simulink library "qs_model"  (R2016a)
settings: Solver=ode45  StartTime=0.0  StopTime=10.0  RelTol=1e-3
values from neighbouring files (symbols this model uses):
  step_time = 0.005    [initialize_variables_kuramoto.m]
libraries: simulink x2
settings Model: Creator=Kundan Panta  LastModifiedBy=Kundan Panta
settings DataIOCC: LimitDataPoints=on
settings DebuggingCC: AllowSymbolicDim=off

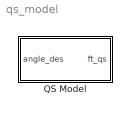
== system qs_model ==
  QS Model : Subsystem

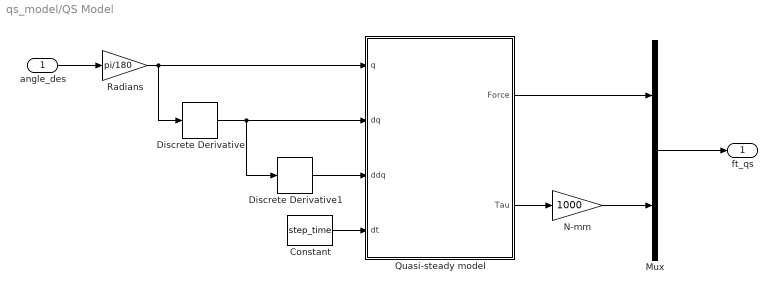
== system qs_model/QS Model ==
  angle_des : Inport  PortDimensions=3
  Constant : Constant  Value=step_time
  Discrete Derivative : simulink/Discrete/Discrete Derivative  gainval=1.0  ICPrevScaledInput=0.0  OutMin=[]  OutMax=[]  OutDataType=fixdt(1, 16)  OutScaling=2^-10  DoSatur=off
  Discrete Derivative1 : simulink/Discrete/Discrete Derivative  gainval=1.0  ICPrevScaledInput=0.0  OutMin=[]  OutMax=[]  OutDataType=fixdt(1, 16)  OutScaling=2^-10  DoSatur=off
  Mux : Mux  Inputs=2
  N-mm : Gain  Gain=1000
  Quasi-steady model : MATLAB Function  TreatAsAtomicUnit=on
  Radians : Gain  Gain=pi/180
  ft_qs : Outport
  wires:
  Quasi-steady model/1(Force) -> Mux/1
  Radians/1 -> Discrete Derivative/1, Quasi-steady model/1(q)
  Quasi-steady model/2(Tau) -> N-mm/1
  Mux/1 -> ft_qs/1
  Constant/1 -> Quasi-steady model/4(dt)
  Discrete Derivative/1 -> Quasi-steady model/2(dq), Discrete Derivative1/1
  angle_des/1 -> Radians/1
  Discrete Derivative1/1 -> Quasi-steady model/3(ddq)
  N-mm/1 -> Mux/2

== matlab function qs_model/QS Model/Quasi-steady model ==
  data: q input; Force output; dq input; ddq input; dt input; Tau output
%#codegen

%%%%%%%%%%%%%%%%%%%%%%%%%%%%%%%%%%%%%%%%%%%%%%%%%%%%%%%%%%%%%%%%%%%%%%%%%%%
%%%%%%%%%%%%%%   Aerodynamic forces and moments calculator   %%%%%%%%%%%%%%
%%%%%%%%%%%%%%%%%%%%%%%%%%%%%%%%%%%%%%%%%%%%%%%%%%%%%%%%%%%%%%%%%%%%%%%%%%%

% This program calcuates the aerodynamic forces and moments generated by a
% flapping wing

% The aerodynamic forces and torques at each wing blade element is
% evaluated by aerodynamics

function [Force,Tau] =Aerodynamic_Force_Torque(q,dq,ddq,dt)
    
% q=[stroke angle;deviation angle; rotation angle]
% dq= dq/dt;
% ddq= dq/dt;

%% Define variables 
    
%     omega_l            % Anular velocity of wing in global frame
%     omega_l_d          % Anular Acc of Right wing in body frame
%     Rcl                %(Rcl* vector_follower=vector_base //    follwer is Wing and Global is base)

    [Rcl,omega_l,omega_l_d] = AngKinZXY(q,dq,ddq);
    %% Hinge parameters

%     lhz  --> Stroke Hinge offset in stroke frame
%     lhx  --> Deviation Hinge offset in deviation frame
%     lhy  --> Rotation Hinge offset in Rotation frame

% Change these parameter according to your setup 
    lhz = [0;0;0];
    lhx = [0;0;0];
    lhy = [0;0.051;0];
    

    vel_h_l = rotz(q(1))*( cross([0;0;dq(1)],lhz) + rotx(q(2))*( cross([dq(2);0;0],lhx) + roty(q(3))*cross([0;dq(3);0],lhy) ));       % Velocity of Hinge in global frame
    
    %% Transform to wing frame
 
    omega_l=Rcl\omega_l;
    omega_l_d=Rcl\omega_l_d;
    vel_h_l  =  Rcl\vel_h_l;
    % transform from global to wing frame



    %%
    rho = 826;      % air density  1.2041(20C) 1.1839(25C)  1.1644(30C)  1.455(35C)
    NumBlade = 10;         % spatial resolution: number of blade elements


% Change these parameter according to your setup 
    Rw = 0.15;          % wing length
    AR = 3;             % Aspect Ratio
    chord = Rw/AR;        % chord length
        

    %% step through a wing span: spanwise location: 0<i<=1
    
    % Initialise variables
    F_t = zeros(3,1);
    Tau_t = zeros(3,1);

    
    for j = 1:NumBlade
        i = j/NumBlade;
        
        % obtain local aerodynamic force/torques in Hinge frame
        % omega_l and omega_r; omega_l_d and omega_r_d in body frame
        % omega_b and vel_h are in global frame
        % omega_b and vel_h have to be expressed differently for left and right wings
        
        % Force and Torque at each blade elements
        [Fi_t, Taui_t] = aerodynamics_left(omega_l,vel_h_l,omega_l_d,i,dt,Rw,chord, NumBlade,rho);

       %% Summation along wing span
       % integrate along wing span and transform to stroke plane frame
       F_t = F_t +  Fi_t;    
       Tau_t =  Tau_t +  Taui_t;


    end

%     % All the forces and torque obtain are in Left and Right Wing frame
%     % Tranform them to Hinge frame 
%  
%     Force=Rcl*F_t;
% 
%     Tau=Rcl*Tau_t ;

    % Keep forces and torques in Wing frame rather than Hinge frame
    Force=F_t;
    Tau=Tau_t;
    
end





%% %%%%%%%%%%%%%%%%%%%%%%%%%%%%%%%%%%%%%%%%%%%%%%%%%%%%%%%%%%%%%%%%%%%%%%%%
%  %%%%%%%%%%%%%%%%%%%%%%%%%%%%%%%%%%%%%%%%%%%%%%%%%%%%%%%%%%%%%%%%%%%%%%%%
%  %%%%%%%%%%%%%%%%%%%%%%%%%%%%%%%%%%%%%%%%%%%%%%%%%%%%%%%%%%%%%%%%%%%%%%%%

%-------------------------------------------------------------------
%----------   Aerodynamics Module For Wing  -------------------
%-------------------------------------------------------------------

% This function takes in wing kinematics (angle/velocity/accleration) and body velocity
% and calcuates the aerodynamic force/torque created by each wing blade (w.r.t local blade coordinate frame)
% then convert it to Hinge frame

% torques are with respect to the wing hinges.

% all the values are w.r.t to local blade coordinate frame (different from stroke
% plane frame), except original input of vel_h, omega_w, omege_w_d and omega_b are in stroke plane frame

% wing coordinate frame: (left wing) x points to ventral side (normal to the wing surface), y from wing base to tip, z from trailing to leading edge

% export tip velocity and span-averaged angle of attack

function [Fi, Taui] = aerodynamics_left(omega_w,vel_h, omega_w_d,i,dt,Rw,chord, NumBlade,rho)
 

%% blade-element analysis 
    % i=location of the blade element
    rle = -i*Rw;  % spanwise location of the blade element
    
    % local wing blade velocity 
    vle = cross(omega_w,[0 rle 0]') + vel_h;            % local leading edge velocity in wing frame
    vle(2)=0;                                                   % igonre radial velocity component                                    

    % angular velocity of the last time instant, here omega_b is assumed to be constant
    omega_wLI = omega_w-omega_w_d*dt;
    
    % velocity of the last time instant
    
    vleLI = cross(omega_wLI,[0 rle 0]') + vel_h;                        
    vleLI(2)=0;                                                 % igonre radial velocity component   
    
    % linear accleration along xw direction
    acc_xw = (vle(1)-vleLI(1))/dt;
    % angualr acceleration about yw direction
    omega_yw_dot = omega_w_d(2);

    
    %% Direction of blade velocity
    % get the direction of the local blade velocity
    if norm(vle) ~= 0
        dir_vle = vle/norm(vle)  ;                 % local leading edge velocity direction vector in left wing frame
        alpha = abs(atan(dir_vle(1)/dir_vle(3)));  
    else
        dir_vle = [0;0;0];
        alpha = 0;  
    end
    
    % local drag direction
    dir_drag = -dir_vle;  
    dir_drag(2)=0; 
    % local lift direction
    dir_lift = roty( -sign( vle(1)) *pi/2 ) * dir_vle;         
    % local angle of attack (consider X as imaginary axis and Z as real axis, only 1st and 2nd quadrants are considered)

    %%  wing sectional lift and drag due to translational force components
    % (2*CD(alpha_l)*rle/R) is sectional drag coefficient
    q   = 0.5*rho*(norm(vle))^2;
    FDi = q*(CD_hu(alpha)) * chord * (Rw/NumBlade)*dir_drag;  
    FLi = q*(CL_hu(alpha)) * chord * (Rw/NumBlade)*dir_lift;

    % center of pressure (translational component)
    r_cof_trans = chord*(0.82*abs(alpha)/pi+0.05);

    %%  wing sectional lift and drag due to rotational force components
    
    % Change these parameter according to your setup 
    x_rot = 0.198;  % rotational axis, 0 corresponds to leading edge
    
    Circulation_rot = pi*(0.75-x_rot) * chord^2 * omega_w(2);  % cirulcation over a wing chord
    F_rot_i = (Rw/NumBlade)*[ rho * Circulation_rot * norm(vle), 0, 0]';
    % center of pressure (rotational component)

    r_cof_rot = x_rot*chord;  % old
    
    %%  wing sectional lift and drag due to added-mass force components
    cr = (-x_rot+0.5)*chord; % distance between center of wing rotation and mid-point of wing chord
    % coefficient of virtual mass
    lamda_x = pi*rho*(0.5*chord)^2;
    lamda_xo = -pi*rho*(0.5*chord)^2*cr;

    % added mass force components
    F_addx_i = lamda_x*acc_xw - lamda_xo*omega_yw_dot;

    % force vector due to added mass
    F_add_i = (Rw/NumBlade)*[F_addx_i, 0,0]'; 

    % center of pressure (added mass component)
    r_cof_add = x_rot*chord;   

    %% summation of all force components and convert them to Hinge frame
    % sum  wing local force vectors
    Fi =  (FDi - FLi -F_add_i - F_rot_i);

    % sum wing local torque vectors
    Taui =(cross([0 rle r_cof_trans]',FDi-FLi) + cross([0 rle r_cof_add]',-F_add_i)+cross([0 rle r_cof_rot]',-F_rot_i));  

 

end


function [R,Omega,alpha] = AngKinZXY(q,dq,ddq)

R=rotz(q(1))*rotx(q(2))*roty(q(3));

w2=[0;0;dq(1)] + rotz(q(1)) * ([dq(2);0;0] );
w1=[0;0;dq(1)] ;

Omega=[0;0;dq(1)]...
    + rotz(q(1)) * [dq(2);0;0] ...
    + rotz(q(1)) * rotx(q(2))*[0;dq(3);0];

alpha=[0;0;ddq(1)]...
    + S(w1)*rotz(q(1)) * [dq(2);0;0] +  rotz(q(1)) * [ddq(2);0;0] ...
    + S(w2)*(rotz(q(1)) * rotx(q(2)))*[0;dq(3);0] +(rotz(q(1)) * rotx(q(2)))*[0;ddq(3);0];
end

function Sw = S(w)
%%%%%%%%%%%%%%%%%%%%%%%%%%%%%%%%%%%%%%%%%%%%%%%%%%%%%%%%%%%%%%%%%%%%%%%%%%%
% % Calculate Cross Product matrix
% % cross(w,R)--> Sw  *  R
%%%%%%%%%%%%%%%%%%%%%%%%%%%%%%%%%%%%%%%%%%%%%%%%%%%%%%%%%%%%%%%%%%%%%%%%%%%
Sw = [0 -w(3) w(2);
    w(3) 0 -w(1);
    -w(2) w(1) 0];
end

function CL = CL_hu(alpha)
alphadeg = alpha *180/pi;       % to degrees
CL = 0.245 + 1.63*sin((2.34*alphadeg - 6.3)*pi/180);
end

function CD = CD_hu(alpha)
alphadeg = alpha *180/pi;       % to degrees
CD = 1.88-1.70*cos((2.27*alphadeg - 10.66)*pi/180);
end

% rotation matrices
% b/c code generation doesn't seem to support built-in ones
function R = rotx(angle)
R = [1 0 0;
    0 cos(angle) -sin(angle);
    0 sin(angle) cos(angle)];
end

function R = roty(angle)
R = [cos(angle) 0 sin(angle);
    0 1 0;
    -sin(angle) 0 cos(angle)];
end

function R = rotz(angle)
R = [cos(angle) -sin(angle) 0;
    sin(angle) cos(angle) 0;
    0 0 1];
end
